simulink model "ej2"  (R2021a)
settings: Solver=VariableStepAuto  StartTime=0.0  StopTime=50  RelTol=1e-3
values from neighbouring files (symbols this model uses):
  g = 9.8    [codigo.m]
  k = 1    [codigo.m]
  m1 = 1    [codigo.m]
  m2 = 0.5    [codigo.m]
  mu = 0.02    [codigo.m]
settings Model: Creator=34622  LastModifiedBy=34622

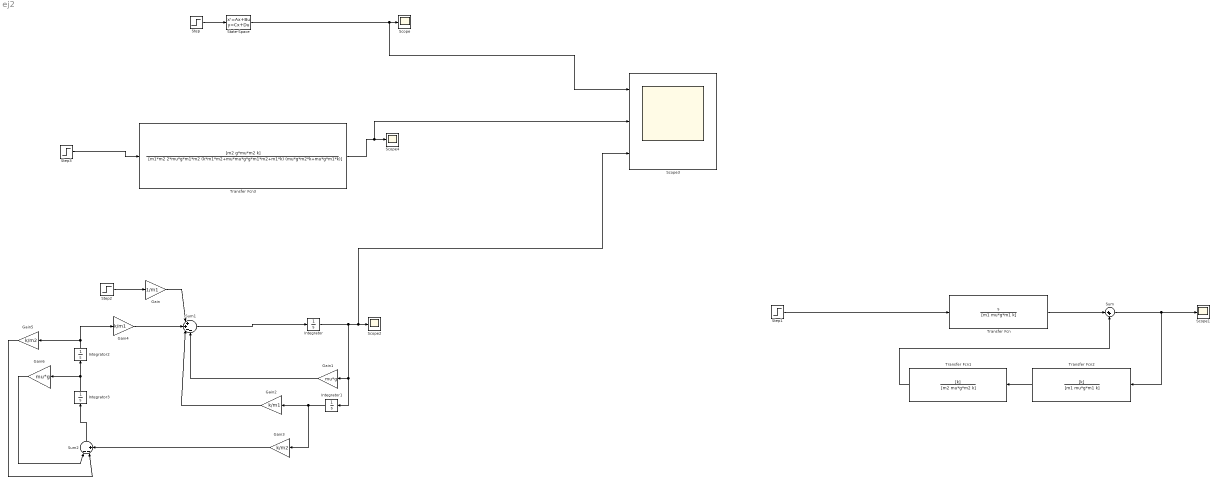
== system ej2 ==
  Gain : Gain  Gain=1/m1
  Gain1 : Gain  Gain=mu*g
  Gain2 : Gain  Gain=k/m1
  Gain3 : Gain  Gain=k/m2
  Gain4 : Gain  Gain=k/m1
  Gain5 : Gain  Gain=k/m2
  Gain6 : Gain  Gain=mu*g
  Integrator{,1..3} (4 alike) : Integrator
  Scope{,1..2,4} (4 alike) : Scope
  Scope3 : Scope  NumInputPorts=3
  State-Space : StateSpace  A=[ 0 1 0 0 ; -k/m1 -mu*g k/m1 0 ;0 0 0 1 ; k/m2 0 -k/m2 -mu*g ]  B=[ 0 ; 1/m1 ; 0 ; 0 ]  C=[0 1 0 0]  D=0  InitialCondition=0
  Step{,1..3} (4 alike) : Step  Time=0  SampleTime=0
  Sum : Sum  Inputs=|++
  Sum1 : Sum  Inputs=|++--
  Sum2 : Sum  Inputs=|--+
  Transfer Fcn : TransferFcn  Numerator=[1 0]  Denominator=[m1 mu*g*m1 k]
  Transfer Fcn1 : TransferFcn  Numerator=[k]  Denominator=[m2 mu*g*m2 k]
  Transfer Fcn2 : TransferFcn  Numerator=[k]  Denominator=[m1 mu*g*m1 k]
  Transfer Fcn3 : TransferFcn  Numerator=[m2 g*mu*m2 k]  Denominator=[m1*m2 2*mu*g*m1*m2 (k*m1*m2+mu*mu*g*g*m1*m2+m1*k) (mu*g*m2*k+mu*g*m1*k)]
  wires:
  Step/1 -> State-Space/1
  State-Space/1 -> Scope3/1, Scope/1
  Transfer Fcn/1 -> Sum/1
  Step1/1 -> Transfer Fcn/1
  Sum/1 -> Transfer Fcn2/1, Scope1/1
  Transfer Fcn1/1 -> Sum/2
  Transfer Fcn2/1 -> Transfer Fcn1/1
  Step2/1 -> Gain/1
  Gain/1 -> Sum1/1
  Sum1/1 -> Integrator/1
  Integrator/1 -> Integrator1/1, Gain1/1, Scope3/3, Scope2/1
  Gain1/1 -> Sum1/4
  Integrator1/1 -> Gain3/1, Gain2/1
  Gain2/1 -> Sum1/3
  Gain4/1 -> Sum1/2
  Integrator2/1 -> Gain5/1, Gain4/1
  Integrator3/1 -> Gain6/1, Integrator2/1
  Sum2/1 -> Integrator3/1
  Gain3/1 -> Sum2/3
  Gain6/1 -> Sum2/1
  Gain5/1 -> Sum2/2
  Step3/1 -> Transfer Fcn3/1
  Transfer Fcn3/1 -> Scope3/2, Scope4/1
